simulink model "sgMdl_BMTS_SimpleVoltageControlWithBCE"  (R2024b)
settings: Solver=FixedStepAuto  StartTime=0.0  StopTime=inf  RelTol=1e-3  EnableMultiTasking=on
undefined symbols (not defined in the file): BCE12, BCE_Set_init, Device_01, sg_bce
libraries: slrealtimeethercatlib x99, simulink x13, slrealtimeutilitieslib x12, SignalEditorBlockLib x1
Description:
  | BMTS - Simple Voltage Control with BCE
settings Model: ModifiedByFormat=Speedgoat  SimulationMode=external  ExtModeTrigDuration=100000  Creator=Speedgoat  LastModifiedBy=Speedgoat
settings SolverCC: ConcurrentTasks=on  AlgebraicLoopSolver=TrustRegion  PositivePriorityOrder=on  InsertRTBMode=Never (minimum delay)
settings DataIOCC: SaveFormat=Array  SaveState=on  SignalLoggingName=logsOut
settings OptimizationCC: BlockReduction=off  BooleanDataType=off  OptimizeBlockIOStorage=off  BufferReuse=off  ReuseModelBlockBuffer=off  GlobalBufferReuse=off  ExpressionFolding=off  LocalBlockOutputs=off  InitFltsAndDblsToZero=on  OptimizeDataStoreBuffers=off  BusAssignmentInplaceUpdate=off
settings DebuggingCC: SaveWithParameterizedLinksMsg=none  MergeDetectMultiDrivingBlocksExec=none  CheckExecutionContextPreStartOutputMsg=on  SignalResolutionControl=TryResolveAllWithWarning  TasksWithSamePriorityMsg=none  UnconnectedInputMsg=warning  UnconnectedOutputMsg=warning  UnconnectedLineMsg=warning  SFUnexpectedBacktrackingDiag=warning  SFNoUnconditionalDefaultTransitionDiag=warning  SFExecutionAtInitializationDiag=none  ArithmeticOperatorsInVariantConditions=warning
settings HardwareCC: ProdBitPerLong=64  ProdLongLongMode=on  ProdHWDeviceType=Intel->x86-64 (Linux 64)
settings ModelReferenceCC: EnableRefExpFcnMdlSchedulingChecks=on  PropagateSignalLabelsOutOfModel=off
settings SFSimCC: SimUseLocalCustomCode=off  SimTargetLang=C++
settings RTWCC: Description=Speedgoat Real-Time Target Machine  SystemTargetFile=speedgoat.tlc  TemplateMakefile=slrealtime_default_tmf  RTWUseLocalCustomCode=off  Toolchain=Simulink Real-Time Toolchain  BuildConfiguration=Faster Runs  TargetLang=C++  GPUComputeCapability=3.5  DLArmComputeVersion=19.05
settings CodeAppCC: StateflowObjectComments=on
settings SimulinkRealTimeTargetCC: SubcomponentCodeInterfacePackaging=Reusable function  InstructionSetFMA=off  LogToMDFFile=off  SLRTFileLogMaxRuns=10
settings ConfigComp: CovMetricSettings=dw  CovSaveCumulativeToWorkspaceVar=on  CovSaveSingleToWorkspaceVar=on  CovExternalEMLEnable=off  CovSFcnEnable=off  CovBoundaryAbsTol=1.0e-5

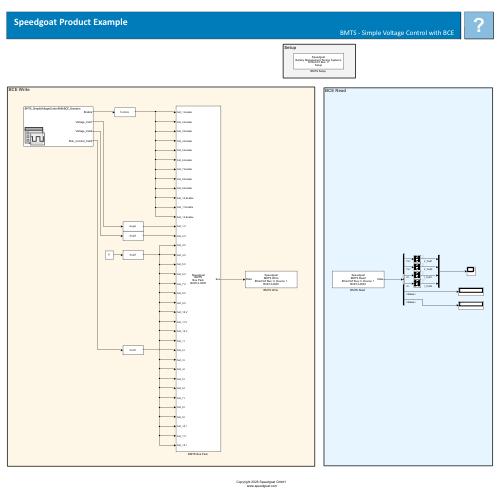
[thumbnail: Simulink's stored preview of the top-level diagram]
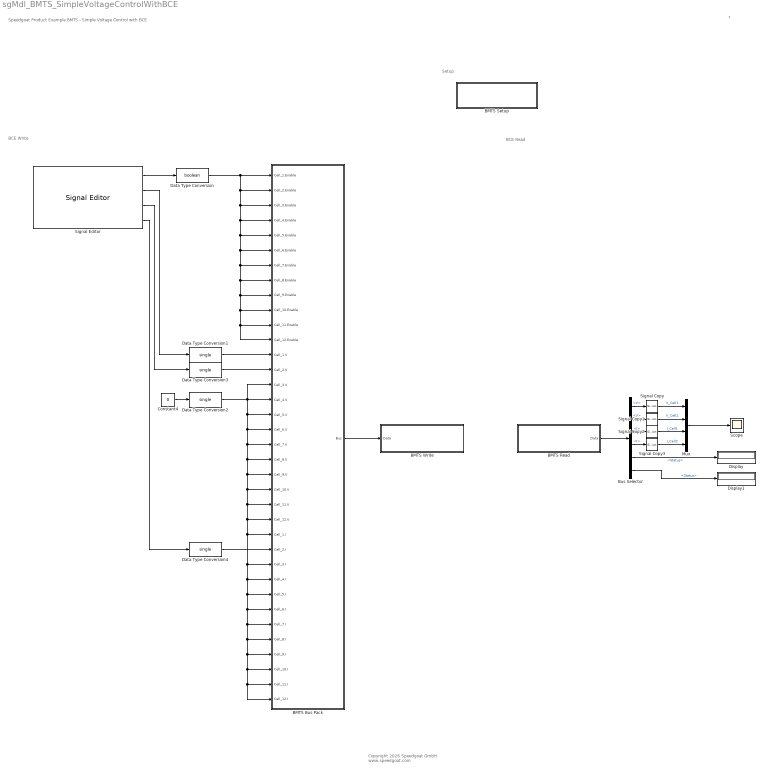
== system sgMdl_BMTS_SimpleVoltageControlWithBCE ==
  note: Setup
  note: BCE Write
  note: BCE Read
  note: Speedgoat Product Example
      | BMTS - Simple Voltage Control with BCE
  note: ?
  note: Copyright 2026 Speedgoat GmbH
      |  www.speedgoat.com
  "BMTS Bus Pack " : Subsystem  mask(bmts_bus_pack){}
      settings: OpenFcn=sg_bce.openFcnBuspack;
      mask Help: eval('sg.utils.help.show(''io_main/refentry_bmts_buspack'');')
      mask Display: disp('Speedgoat\nBMTS\nBus Pack\nBCE12-0605');
  "BMTS Read " : Subsystem  InitFcn=sg_bce.checkNumberOfBlocksGlobal(bdroot);  mask(bce_read){}
      settings: OpenFcn=sg_bce.openFcnRead;
      mask Help: eval('sg.utils.help.show(''io_main/refentry_bce_read'');')
      mask Display: disp('Speedgoat\nBMTS Read\nEtherCAT Bus: 0, Device: 1\nBCE12-0605');port_label('output',1,'Data');
  "BMTS Setup " : Subsystem  LoadFcn=|  InitFcn=|  mask(bce_setup){}
      LoadFcn=|
      | sg_bce.createBusSignals;
      | sg_bce.setupEniCallback(gcb, bdroot);
      InitFcn=|
      | sg_bce.createBusSignals;
      | sg_bce.checkNumberOfBlocksGlobal(bdroot);
      | sg_bce.setupEniCallback(gcb, bdroot);
      settings: OpenFcn=sg_bce.openFcnSetup;
      mask Help: eval('sg.utils.help.show(''io_main/refentry_bce_setup'');')
      mask Display: disp('Speedgoat\nBattery Management Testing Systems\nEtherCAT Bus: 0\nSetup');
  "BMTS Write " : Subsystem  InitFcn=sg_bce.checkNumberOfBlocksGlobal(bdroot);  mask(bce_write){}
      settings: OpenFcn=sg_bce.openFcnWrite;
      mask Help: eval('sg.utils.help.show(''io_main/refentry_bce_write'');')
      mask Display: disp('Speedgoat\nBMTS Write\nEtherCAT Bus: 0, Device: 1\nBCE12-0605');port_label('input',1,'Data');
  Bus Selector : BusSelector  OutputSignals=Cell_1.V,Cell_2.V,Cell_1.I,Cell_2.I,Cell_1.Status,Cell_2.Status
  Constant4 : Constant  Value=0
  Data Type Conversion : DataTypeConversion  OutDataTypeStr=boolean  SaturateOnIntegerOverflow=off  RndMeth=Floor
  Data Type Conversion{1..4} (4 alike) : DataTypeConversion  OutDataTypeStr=single  SaturateOnIntegerOverflow=off  RndMeth=Floor
  Display : Display
  Display1 : Display
  Mux : Mux
  Scope : Scope
  Signal Copy{,1..3} (4 alike) : SignalConversion  OverrideOpt=off
  Signal Editor : SignalEditorBlockLib/Signal Editor  FileName=BMTS_SimpleVoltageControlWithBCE_Scenario.mat  ActiveScenario=BMTS_SimpleVoltageControlWithBCE_Scenario  ActiveSignal=Voltage_Cell2  IsBus=off  OutputBusObjectStr=Bus: BusObject  SampleTime=0  ZeroCross=off  OutputAfterFinalValue=Setting to zero  Unit=inherit  PreserveSignalName=on  ApplySigPropsToAllScenarios=on  ApplySigPropsToAllSignals=off
  wires:
  Signal Editor/2 -> Data Type Conversion1/1
  "BMTS Bus Pack "/1(Bus) -> "BMTS Write "/1(Data)
  Signal Editor/1 -> Data Type Conversion/1
  "BMTS Read "/1(Data) -> Bus Selector/1
  Data Type Conversion/1 -> "BMTS Bus Pack "/11(Cell_11.Enable), "BMTS Bus Pack "/12(Cell_12.Enable), "BMTS Bus Pack "/10(Cell_10.Enable), "BMTS Bus Pack "/9(Cell_9.Enable), "BMTS Bus Pack "/8(Cell_8.Enable), "BMTS Bus Pack "/7(Cell_7.Enable), "BMTS Bus Pack "/6(Cell_6.Enable), "BMTS Bus Pack "/5(Cell_5.Enable), "BMTS Bus Pack "/4(Cell_4.Enable), "BMTS Bus Pack "/3(Cell_3.Enable), "BMTS Bus Pack "/2(Cell_2.Enable), "BMTS Bus Pack "/1(Cell_1.Enable)
  Constant4/1 -> Data Type Conversion2/1
  Data Type Conversion1/1 -> "BMTS Bus Pack "/13(Cell_1.V)
  Data Type Conversion2/1 -> "BMTS Bus Pack "/35(Cell_11.I), "BMTS Bus Pack "/36(Cell_12.I), "BMTS Bus Pack "/34(Cell_10.I), "BMTS Bus Pack "/33(Cell_9.I), "BMTS Bus Pack "/32(Cell_8.I), "BMTS Bus Pack "/31(Cell_7.I), "BMTS Bus Pack "/30(Cell_6.I), "BMTS Bus Pack "/29(Cell_5.I), "BMTS Bus Pack "/28(Cell_4.I), "BMTS Bus Pack "/27(Cell_3.I), "BMTS Bus Pack "/25(Cell_1.I), "BMTS Bus Pack "/24(Cell_12.V), "BMTS Bus Pack "/23(Cell_11.V), "BMTS Bus Pack "/22(Cell_10.V), "BMTS Bus Pack "/21(Cell_9.V), "BMTS Bus Pack "/20(Cell_8.V), "BMTS Bus Pack "/19(Cell_7.V), "BMTS Bus Pack "/18(Cell_6.V), "BMTS Bus Pack "/17(Cell_5.V), "BMTS Bus Pack "/16(Cell_4.V), "BMTS Bus Pack "/15(Cell_3.V)
  Bus Selector/1 -> Signal Copy/1  "<V>"
  Bus Selector/2 -> Signal Copy1/1  "<V>"
  Bus Selector/3 -> Signal Copy2/1  "<I>"
  Bus Selector/4 -> Signal Copy3/1  "<I>"
  Bus Selector/5 -> Display/1  "<Status>"
  Bus Selector/6 -> Display1/1  "<Status>"
  Signal Copy/1 -> Mux/1  "V_Cell1"
  Signal Copy1/1 -> Mux/2  "V_Cell2"
  Signal Copy2/1 -> Mux/3  "I_Cell1"
  Signal Copy3/1 -> Mux/4  "I_Cell2"
  Data Type Conversion3/1 -> "BMTS Bus Pack "/14(Cell_2.V)
  Signal Editor/3 -> Data Type Conversion3/1
  Signal Editor/4 -> Data Type Conversion4/1
  Data Type Conversion4/1 -> "BMTS Bus Pack "/26(Cell_2.I)
  Mux/1 -> Scope/1

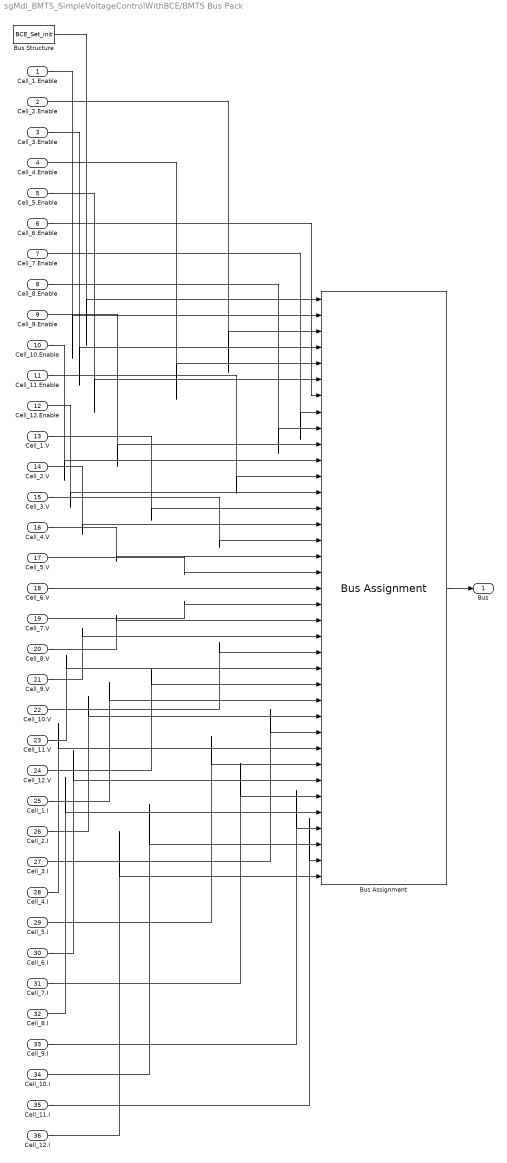
== system sgMdl_BMTS_SimpleVoltageControlWithBCE/BMTS Bus Pack  ==
  Cell_1.Enable : Inport
  Cell_2.Enable : Inport  Port=2
  Cell_3.Enable : Inport  Port=3
  Cell_4.Enable : Inport  Port=4
  Cell_5.Enable : Inport  Port=5
  Cell_6.Enable : Inport  Port=6
  Cell_7.Enable : Inport  Port=7
  Cell_8.Enable : Inport  Port=8
  Cell_9.Enable : Inport  Port=9
  Cell_10.Enable : Inport  Port=10
  Cell_11.Enable : Inport  Port=11
  Cell_12.Enable : Inport  Port=12
  Cell_1.V : Inport  Port=13
  Cell_2.V : Inport  Port=14
  Cell_3.V : Inport  Port=15
  Cell_4.V : Inport  Port=16
  Cell_5.V : Inport  Port=17
  Cell_6.V : Inport  Port=18
  Cell_7.V : Inport  Port=19
  Cell_8.V : Inport  Port=20
  Cell_9.V : Inport  Port=21
  Cell_10.V : Inport  Port=22
  Cell_11.V : Inport  Port=23
  Cell_12.V : Inport  Port=24
  Cell_1.I : Inport  Port=25
  Cell_2.I : Inport  Port=26
  Cell_3.I : Inport  Port=27
  Cell_4.I : Inport  Port=28
  Cell_5.I : Inport  Port=29
  Cell_6.I : Inport  Port=30
  Cell_7.I : Inport  Port=31
  Cell_8.I : Inport  Port=32
  Cell_9.I : Inport  Port=33
  Cell_10.I : Inport  Port=34
  Cell_11.I : Inport  Port=35
  Cell_12.I : Inport  Port=36
  Bus Assignment : BusAssignment  AssignedSignals=Cell_1.Enable,Cell_2.Enable,Cell_3.Enable,Cell_4.Enable,Cell_5.Enable,Cell_6.Enable,Cell_7.Enable,Cell_8.Enable,Cell_9.Enable,Cell_10.Enable,Cell_11.Enable,Cell_12.Enable,Cell_1.V,Cell_2.V,Cell_3.V,Cell_4.V,Cell_5.V,Cell_6.V,Cell_7.V,Cell_8.V,Cell_9.V,Cell_10.V,Cell_11.V,Cell_12.V,Cell_1.I,Cell_2.I,Cell_3.I,Cell_4.I,Cell_5.I,Cell_6.I,Cell_7.I,Cell_8.I,Cell_9.I,Cell_10.I,Cell_11.I,Cell_12.I
  Bus Structure : Constant  Value=BCE_Set_init  OutDataTypeStr=Bus: BCE_Set
  Bus : Outport
  wires:
  Cell_3.Enable/1 -> Bus Assignment/4
  Cell_5.Enable/1 -> Bus Assignment/6
  Cell_1.I/1 -> Bus Assignment/26
  Bus Structure/1 -> Bus Assignment/1
  Cell_1.Enable/1 -> Bus Assignment/2
  Cell_8.I/1 -> Bus Assignment/33
  Cell_7.Enable/1 -> Bus Assignment/8
  Cell_9.I/1 -> Bus Assignment/34
  Cell_2.Enable/1 -> Bus Assignment/3
  Cell_5.V/1 -> Bus Assignment/18
  Cell_4.Enable/1 -> Bus Assignment/5
  Cell_3.V/1 -> Bus Assignment/16
  Cell_8.Enable/1 -> Bus Assignment/9
  Cell_6.Enable/1 -> Bus Assignment/7
  Cell_6.I/1 -> Bus Assignment/31
  Cell_9.Enable/1 -> Bus Assignment/10
  Cell_10.Enable/1 -> Bus Assignment/11
  Cell_11.Enable/1 -> Bus Assignment/12
  Cell_11.I/1 -> Bus Assignment/36
  Cell_12.Enable/1 -> Bus Assignment/13
  Cell_1.V/1 -> Bus Assignment/14
  Cell_2.V/1 -> Bus Assignment/15
  Cell_12.V/1 -> Bus Assignment/25
  Cell_4.V/1 -> Bus Assignment/17
  Cell_6.V/1 -> Bus Assignment/19
  Cell_7.V/1 -> Bus Assignment/20
  Cell_3.I/1 -> Bus Assignment/28
  Cell_8.V/1 -> Bus Assignment/21
  Cell_9.V/1 -> Bus Assignment/22
  Cell_10.V/1 -> Bus Assignment/23
  Cell_11.V/1 -> Bus Assignment/24
  Cell_2.I/1 -> Bus Assignment/27
  Cell_4.I/1 -> Bus Assignment/29
  Cell_5.I/1 -> Bus Assignment/30
  Cell_7.I/1 -> Bus Assignment/32
  Cell_10.I/1 -> Bus Assignment/35
  Cell_12.I/1 -> Bus Assignment/37
  Bus Assignment/1 -> Bus/1

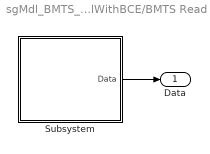
== system sgMdl_BMTS_SimpleVoltageControlWithBCE/BMTS Read  ==
  Subsystem : Subsystem
  Data : Outport  OutDataTypeStr=Bus: BCE_Get
  wires:
  Subsystem/1(Data) -> Data/1

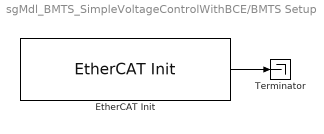
== system sgMdl_BMTS_SimpleVoltageControlWithBCE/BMTS Setup  ==
  EtherCAT Init : slrealtimeethercatlib/EtherCAT Init  Priority=0  config_file=C:\Users\timo.straessle\AppData\Local\Temp\sg_bmts\sgMdl_BMTS_SimpleVoltageControlWithBCE\sg_bmts_ENI_bus0.xml  device_id=0  portnum=1  initstate=2  dctuning=0  enaDebug=0  logFile='c:\dbglog.txt'  sample_time=0.001000  DCMode=0
  Terminator : Terminator
  wires:
  EtherCAT Init/1 -> Terminator/1

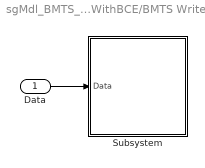
== system sgMdl_BMTS_SimpleVoltageControlWithBCE/BMTS Write  ==
  Data : Inport  OutDataTypeStr=Bus: BCE_Set
  Subsystem : Subsystem
  wires:
  Data/1 -> Subsystem/1(Data)

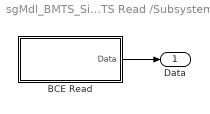
== system sgMdl_BMTS_SimpleVoltageControlWithBCE/BMTS Read /Subsystem ==
  "BCE Read " : Subsystem
  Data : Outport  OutDataTypeStr=Bus: BCE_Get
  wires:
  "BCE Read "/1(Data) -> Data/1

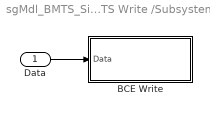
== system sgMdl_BMTS_SimpleVoltageControlWithBCE/BMTS Write /Subsystem ==
  Data : Inport  OutDataTypeStr=Bus: BCE_Set
  "BCE Write " : Subsystem
  wires:
  Data/1 -> "BCE Write "/1(Data)

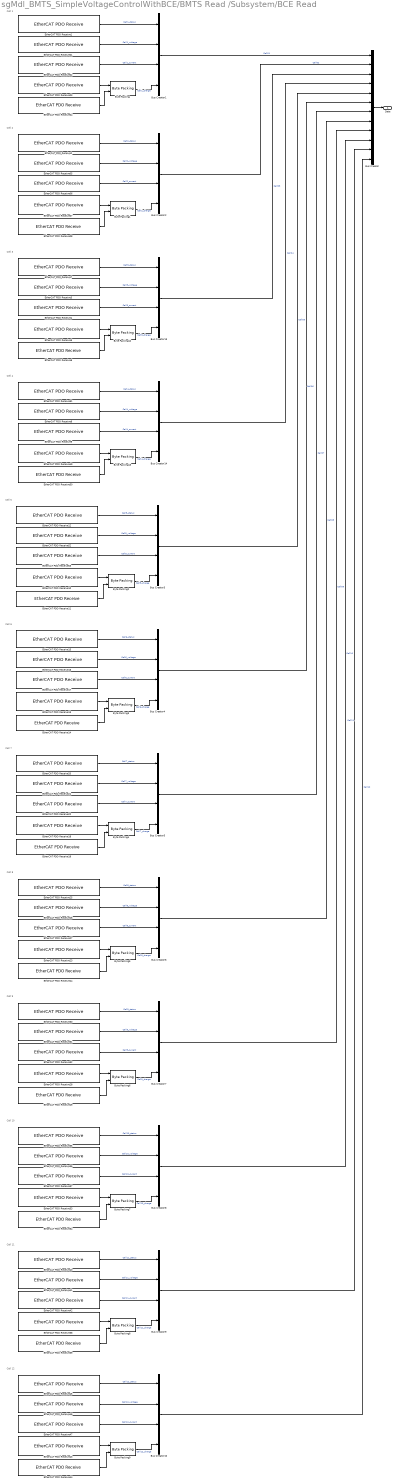
== system sgMdl_BMTS_SimpleVoltageControlWithBCE/BMTS Read /Subsystem/BCE Read  ==
  note: Cell 7
  note: Cell 2
  note: Cell 6
  note: Cell 8
  note: Cell 12
  note: Cell 11
  note: Cell 3
  note: Cell 5
  note: Cell 4
  note: Cell 10
  note: Cell 9
  note: Cell 1
  Bus Creator : BusCreator  Inputs=12  OutDataTypeStr=Bus: BCE_Get
      settings: InheritFromInputs=off
  Bus Creator{1..10,13..14} (12 alike) : BusCreator  Inputs=4  OutDataTypeStr=Bus: Cell_Get
      settings: InheritFromInputs=off
  Byte Packing{,1..9,12..13} (12 alike) : slrealtimeutilitieslib/Byte Packing  MaskPackedDataType=uint64  MaskUnpackedDataTypes={'uint32','uint32'}  MaskAlignment=1
  EtherCAT PDO Receive01 : slrealtimeethercatlib/EtherCAT PDO Receive  Priority=2  sig_name=Device_01 (BCE12-0605).Tx_Cell_01.voltage  sig_offset=16  sig_type=single  type_size=32  sig_dim=1  device_id=0  sample_time=0.001000
  EtherCAT PDO Receive02 : slrealtimeethercatlib/EtherCAT PDO Receive  Priority=2  sig_name=Device_01 (BCE12-0605).Tx_Cell_01.current  sig_offset=48  sig_type=single  type_size=32  sig_dim=1  device_id=0  sample_time=0.001000
  EtherCAT PDO Receive03 : slrealtimeethercatlib/EtherCAT PDO Receive  Priority=2  sig_name=Device_01 (BCE12-0605).Tx_Cell_01.chargeMSB  sig_offset=80  sig_type=uint32  type_size=32  sig_dim=1  device_id=0  sample_time=0.001000
  EtherCAT PDO Receive04 : slrealtimeethercatlib/EtherCAT PDO Receive  Priority=2  sig_name=Device_01 (BCE12-0605).Tx_Cell_01.chargeLSB  sig_offset=112  sig_type=uint32  type_size=32  sig_dim=1  device_id=0  sample_time=0.001000
  EtherCAT PDO Receive05 : slrealtimeethercatlib/EtherCAT PDO Receive  Priority=2  sig_name=Device_01 (BCE12-0605).Tx_Cell_02.voltage  sig_offset=160  sig_type=single  type_size=32  sig_dim=1  device_id=0  sample_time=0.001000
  EtherCAT PDO Receive06 : slrealtimeethercatlib/EtherCAT PDO Receive  Priority=2  sig_name=Device_01 (BCE12-0605).Tx_Cell_02.current  sig_offset=192  sig_type=single  type_size=32  sig_dim=1  device_id=0  sample_time=0.001000
  EtherCAT PDO Receive07 : slrealtimeethercatlib/EtherCAT PDO Receive  Priority=2  sig_name=Device_01 (BCE12-0605).Tx_Cell_02.chargeMSB  sig_offset=224  sig_type=uint32  type_size=32  sig_dim=1  device_id=0  sample_time=0.001000
  EtherCAT PDO Receive08 : slrealtimeethercatlib/EtherCAT PDO Receive  Priority=2  sig_name=Device_01 (BCE12-0605).Tx_Cell_02.chargeLSB  sig_offset=256  sig_type=uint32  type_size=32  sig_dim=1  device_id=0  sample_time=0.001000
  EtherCAT PDO Receive1 : slrealtimeethercatlib/EtherCAT PDO Receive  Priority=2  sig_name=Device_01 (BCE12-0605).Tx_Cell_01.status  sig_offset=0  sig_type=uint16  type_size=16  sig_dim=1  device_id=0  sample_time=0.001000
  EtherCAT PDO Receive10 : slrealtimeethercatlib/EtherCAT PDO Receive  Priority=2  sig_name=Device_01 (BCE12-0605).Tx_Cell_05.chargeMSB  sig_offset=656  sig_type=uint32  type_size=32  sig_dim=1  device_id=0  sample_time=0.001000
  EtherCAT PDO Receive11 : slrealtimeethercatlib/EtherCAT PDO Receive  Priority=2  sig_name=Device_01 (BCE12-0605).Tx_Cell_05.chargeLSB  sig_offset=688  sig_type=uint32  type_size=32  sig_dim=1  device_id=0  sample_time=0.001000
  EtherCAT PDO Receive12 : slrealtimeethercatlib/EtherCAT PDO Receive  Priority=2  sig_name=Device_01 (BCE12-0605).Tx_Cell_05.status  sig_offset=576  sig_type=uint16  type_size=16  sig_dim=1  device_id=0  sample_time=0.001000
  EtherCAT PDO Receive13 : slrealtimeethercatlib/EtherCAT PDO Receive  Priority=2  sig_name=Device_01 (BCE12-0605).Tx_Cell_06.chargeMSB  sig_offset=800  sig_type=uint32  type_size=32  sig_dim=1  device_id=0  sample_time=0.001000
  EtherCAT PDO Receive14 : slrealtimeethercatlib/EtherCAT PDO Receive  Priority=2  sig_name=Device_01 (BCE12-0605).Tx_Cell_06.chargeLSB  sig_offset=832  sig_type=uint32  type_size=32  sig_dim=1  device_id=0  sample_time=0.001000
  EtherCAT PDO Receive15 : slrealtimeethercatlib/EtherCAT PDO Receive  Priority=2  sig_name=Device_01 (BCE12-0605).Tx_Cell_06.status  sig_offset=720  sig_type=uint16  type_size=16  sig_dim=1  device_id=0  sample_time=0.001000
  EtherCAT PDO Receive16 : slrealtimeethercatlib/EtherCAT PDO Receive  Priority=2  sig_name=Device_01 (BCE12-0605).Tx_Cell_06.voltage  sig_offset=736  sig_type=single  type_size=32  sig_dim=1  device_id=0  sample_time=0.001000
  EtherCAT PDO Receive17 : slrealtimeethercatlib/EtherCAT PDO Receive  Priority=2  sig_name=Device_01 (BCE12-0605).Tx_Cell_06.current  sig_offset=768  sig_type=single  type_size=32  sig_dim=1  device_id=0  sample_time=0.001000
  EtherCAT PDO Receive18 : slrealtimeethercatlib/EtherCAT PDO Receive  Priority=2  sig_name=Device_01 (BCE12-0605).Tx_Cell_07.chargeMSB  sig_offset=944  sig_type=uint32  type_size=32  sig_dim=1  device_id=0  sample_time=0.001000
  EtherCAT PDO Receive19 : slrealtimeethercatlib/EtherCAT PDO Receive  Priority=2  sig_name=Device_01 (BCE12-0605).Tx_Cell_07.chargeLSB  sig_offset=976  sig_type=uint32  type_size=32  sig_dim=1  device_id=0  sample_time=0.001000
  EtherCAT PDO Receive2 : slrealtimeethercatlib/EtherCAT PDO Receive  Priority=2  sig_name=Device_01 (BCE12-0605).Tx_Cell_02.status  sig_offset=144  sig_type=uint16  type_size=16  sig_dim=1  device_id=0  sample_time=0.001000
  EtherCAT PDO Receive20 : slrealtimeethercatlib/EtherCAT PDO Receive  Priority=2  sig_name=Device_01 (BCE12-0605).Tx_Cell_07.status  sig_offset=864  sig_type=uint16  type_size=16  sig_dim=1  device_id=0  sample_time=0.001000
  EtherCAT PDO Receive21 : slrealtimeethercatlib/EtherCAT PDO Receive  Priority=2  sig_name=Device_01 (BCE12-0605).Tx_Cell_07.voltage  sig_offset=880  sig_type=single  type_size=32  sig_dim=1  device_id=0  sample_time=0.001000
  EtherCAT PDO Receive22 : slrealtimeethercatlib/EtherCAT PDO Receive  Priority=2  sig_name=Device_01 (BCE12-0605).Tx_Cell_07.current  sig_offset=912  sig_type=single  type_size=32  sig_dim=1  device_id=0  sample_time=0.001000
  EtherCAT PDO Receive23 : slrealtimeethercatlib/EtherCAT PDO Receive  Priority=2  sig_name=Device_01 (BCE12-0605).Tx_Cell_08.chargeMSB  sig_offset=1088  sig_type=uint32  type_size=32  sig_dim=1  device_id=0  sample_time=0.001000
  EtherCAT PDO Receive24 : slrealtimeethercatlib/EtherCAT PDO Receive  Priority=2  sig_name=Device_01 (BCE12-0605).Tx_Cell_08.chargeLSB  sig_offset=1120  sig_type=uint32  type_size=32  sig_dim=1  device_id=0  sample_time=0.001000
  EtherCAT PDO Receive25 : slrealtimeethercatlib/EtherCAT PDO Receive  Priority=2  sig_name=Device_01 (BCE12-0605).Tx_Cell_08.status  sig_offset=1008  sig_type=uint16  type_size=16  sig_dim=1  device_id=0  sample_time=0.001000
  EtherCAT PDO Receive26 : slrealtimeethercatlib/EtherCAT PDO Receive  Priority=2  sig_name=Device_01 (BCE12-0605).Tx_Cell_08.voltage  sig_offset=1024  sig_type=single  type_size=32  sig_dim=1  device_id=0  sample_time=0.001000
  EtherCAT PDO Receive27 : slrealtimeethercatlib/EtherCAT PDO Receive  Priority=2  sig_name=Device_01 (BCE12-0605).Tx_Cell_08.current  sig_offset=1056  sig_type=single  type_size=32  sig_dim=1  device_id=0  sample_time=0.001000
  EtherCAT PDO Receive28 : slrealtimeethercatlib/EtherCAT PDO Receive  Priority=2  sig_name=Device_01 (BCE12-0605).Tx_Cell_09.chargeMSB  sig_offset=1232  sig_type=uint32  type_size=32  sig_dim=1  device_id=0  sample_time=0.001000
  EtherCAT PDO Receive29 : slrealtimeethercatlib/EtherCAT PDO Receive  Priority=2  sig_name=Device_01 (BCE12-0605).Tx_Cell_09.chargeLSB  sig_offset=1264  sig_type=uint32  type_size=32  sig_dim=1  device_id=0  sample_time=0.001000
  EtherCAT PDO Receive3 : slrealtimeethercatlib/EtherCAT PDO Receive  Priority=2  sig_name=Device_01 (BCE12-0605).Tx_Cell_03.voltage  sig_offset=304  sig_type=single  type_size=32  sig_dim=1  device_id=0  sample_time=0.001000
  EtherCAT PDO Receive30 : slrealtimeethercatlib/EtherCAT PDO Receive  Priority=2  sig_name=Device_01 (BCE12-0605).Tx_Cell_09.status  sig_offset=1152  sig_type=uint16  type_size=16  sig_dim=1  device_id=0  sample_time=0.001000
  EtherCAT PDO Receive31 : slrealtimeethercatlib/EtherCAT PDO Receive  Priority=2  sig_name=Device_01 (BCE12-0605).Tx_Cell_09.voltage  sig_offset=1168  sig_type=single  type_size=32  sig_dim=1  device_id=0  sample_time=0.001000
  EtherCAT PDO Receive32 : slrealtimeethercatlib/EtherCAT PDO Receive  Priority=2  sig_name=Device_01 (BCE12-0605).Tx_Cell_09.current  sig_offset=1200  sig_type=single  type_size=32  sig_dim=1  device_id=0  sample_time=0.001000
  EtherCAT PDO Receive33 : slrealtimeethercatlib/EtherCAT PDO Receive  Priority=2  sig_name=Device_01 (BCE12-0605).Tx_Cell_10.chargeMSB  sig_offset=1376  sig_type=uint32  type_size=32  sig_dim=1  device_id=0  sample_time=0.001000
  EtherCAT PDO Receive34 : slrealtimeethercatlib/EtherCAT PDO Receive  Priority=2  sig_name=Device_01 (BCE12-0605).Tx_Cell_10.chargeLSB  sig_offset=1408  sig_type=uint32  type_size=32  sig_dim=1  device_id=0  sample_time=0.001000
  EtherCAT PDO Receive35 : slrealtimeethercatlib/EtherCAT PDO Receive  Priority=2  sig_name=Device_01 (BCE12-0605).Tx_Cell_10.status  sig_offset=1296  sig_type=uint16  type_size=16  sig_dim=1  device_id=0  sample_time=0.001000
  EtherCAT PDO Receive36 : slrealtimeethercatlib/EtherCAT PDO Receive  Priority=2  sig_name=Device_01 (BCE12-0605).Tx_Cell_10.voltage  sig_offset=1312  sig_type=single  type_size=32  sig_dim=1  device_id=0  sample_time=0.001000
  EtherCAT PDO Receive37 : slrealtimeethercatlib/EtherCAT PDO Receive  Priority=2  sig_name=Device_01 (BCE12-0605).Tx_Cell_10.current  sig_offset=1344  sig_type=single  type_size=32  sig_dim=1  device_id=0  sample_time=0.001000
  EtherCAT PDO Receive38 : slrealtimeethercatlib/EtherCAT PDO Receive  Priority=2  sig_name=Device_01 (BCE12-0605).Tx_Cell_11.chargeMSB  sig_offset=1520  sig_type=uint32  type_size=32  sig_dim=1  device_id=0  sample_time=0.001000
  EtherCAT PDO Receive39 : slrealtimeethercatlib/EtherCAT PDO Receive  Priority=2  sig_name=Device_01 (BCE12-0605).Tx_Cell_11.chargeLSB  sig_offset=1552  sig_type=uint32  type_size=32  sig_dim=1  device_id=0  sample_time=0.001000
  EtherCAT PDO Receive4 : slrealtimeethercatlib/EtherCAT PDO Receive  Priority=2  sig_name=Device_01 (BCE12-0605).Tx_Cell_03.current  sig_offset=336  sig_type=single  type_size=32  sig_dim=1  device_id=0  sample_time=0.001000
  EtherCAT PDO Receive40 : slrealtimeethercatlib/EtherCAT PDO Receive  Priority=2  sig_name=Device_01 (BCE12-0605).Tx_Cell_11.status  sig_offset=1440  sig_type=uint16  type_size=16  sig_dim=1  device_id=0  sample_time=0.001000
  EtherCAT PDO Receive41 : slrealtimeethercatlib/EtherCAT PDO Receive  Priority=2  sig_name=Device_01 (BCE12-0605).Tx_Cell_11.voltage  sig_offset=1456  sig_type=single  type_size=32  sig_dim=1  device_id=0  sample_time=0.001000
  EtherCAT PDO Receive42 : slrealtimeethercatlib/EtherCAT PDO Receive  Priority=2  sig_name=Device_01 (BCE12-0605).Tx_Cell_11.current  sig_offset=1488  sig_type=single  type_size=32  sig_dim=1  device_id=0  sample_time=0.001000
  EtherCAT PDO Receive43 : slrealtimeethercatlib/EtherCAT PDO Receive  Priority=2  sig_name=Device_01 (BCE12-0605).Tx_Cell_12.chargeMSB  sig_offset=1664  sig_type=uint32  type_size=32  sig_dim=1  device_id=0  sample_time=0.001000
  EtherCAT PDO Receive44 : slrealtimeethercatlib/EtherCAT PDO Receive  Priority=2  sig_name=Device_01 (BCE12-0605).Tx_Cell_12.chargeLSB  sig_offset=1696  sig_type=uint32  type_size=32  sig_dim=1  device_id=0  sample_time=0.001000
  EtherCAT PDO Receive45 : slrealtimeethercatlib/EtherCAT PDO Receive  Priority=2  sig_name=Device_01 (BCE12-0605).Tx_Cell_12.status  sig_offset=1584  sig_type=uint16  type_size=16  sig_dim=1  device_id=0  sample_time=0.001000
  EtherCAT PDO Receive46 : slrealtimeethercatlib/EtherCAT PDO Receive  Priority=2  sig_name=Device_01 (BCE12-0605).Tx_Cell_12.voltage  sig_offset=1600  sig_type=single  type_size=32  sig_dim=1  device_id=0  sample_time=0.001000
  EtherCAT PDO Receive47 : slrealtimeethercatlib/EtherCAT PDO Receive  Priority=2  sig_name=Device_01 (BCE12-0605).Tx_Cell_12.current  sig_offset=1632  sig_type=single  type_size=32  sig_dim=1  device_id=0  sample_time=0.001000
  EtherCAT PDO Receive49 : slrealtimeethercatlib/EtherCAT PDO Receive  Priority=2  sig_name=Device_01 (BCE12-0605).Tx_Cell_04.chargeMSB  sig_offset=512  sig_type=uint32  type_size=32  sig_dim=1  device_id=0  sample_time=0.001000
  EtherCAT PDO Receive5 : slrealtimeethercatlib/EtherCAT PDO Receive  Priority=2  sig_name=Device_01 (BCE12-0605).Tx_Cell_03.chargeMSB  sig_offset=368  sig_type=uint32  type_size=32  sig_dim=1  device_id=0  sample_time=0.001000
  EtherCAT PDO Receive50 : slrealtimeethercatlib/EtherCAT PDO Receive  Priority=2  sig_name=Device_01 (BCE12-0605).Tx_Cell_04.chargeLSB  sig_offset=544  sig_type=uint32  type_size=32  sig_dim=1  device_id=0  sample_time=0.001000
  EtherCAT PDO Receive51 : slrealtimeethercatlib/EtherCAT PDO Receive  Priority=2  sig_name=Device_01 (BCE12-0605).Tx_Cell_04.status  sig_offset=432  sig_type=uint16  type_size=16  sig_dim=1  device_id=0  sample_time=0.001000
  EtherCAT PDO Receive52 : slrealtimeethercatlib/EtherCAT PDO Receive  Priority=2  sig_name=Device_01 (BCE12-0605).Tx_Cell_05.voltage  sig_offset=592  sig_type=single  type_size=32  sig_dim=1  device_id=0  sample_time=0.001000
  EtherCAT PDO Receive53 : slrealtimeethercatlib/EtherCAT PDO Receive  Priority=2  sig_name=Device_01 (BCE12-0605).Tx_Cell_05.current  sig_offset=624  sig_type=single  type_size=32  sig_dim=1  device_id=0  sample_time=0.001000
  EtherCAT PDO Receive6 : slrealtimeethercatlib/EtherCAT PDO Receive  Priority=2  sig_name=Device_01 (BCE12-0605).Tx_Cell_03.chargeLSB  sig_offset=400  sig_type=uint32  type_size=32  sig_dim=1  device_id=0  sample_time=0.001000
  EtherCAT PDO Receive7 : slrealtimeethercatlib/EtherCAT PDO Receive  Priority=2  sig_name=Device_01 (BCE12-0605).Tx_Cell_03.status  sig_offset=288  sig_type=uint16  type_size=16  sig_dim=1  device_id=0  sample_time=0.001000
  EtherCAT PDO Receive8 : slrealtimeethercatlib/EtherCAT PDO Receive  Priority=2  sig_name=Device_01 (BCE12-0605).Tx_Cell_04.voltage  sig_offset=448  sig_type=single  type_size=32  sig_dim=1  device_id=0  sample_time=0.001000
  EtherCAT PDO Receive9 : slrealtimeethercatlib/EtherCAT PDO Receive  Priority=2  sig_name=Device_01 (BCE12-0605).Tx_Cell_04.current  sig_offset=480  sig_type=single  type_size=32  sig_dim=1  device_id=0  sample_time=0.001000
  Data : Outport  OutDataTypeStr=Bus: BCE_Get
  wires:
  EtherCAT PDO Receive04/1 -> Byte Packing/2
  EtherCAT PDO Receive53/1 -> Bus Creator3/3  "Cell5_current"
  Bus Creator7/1 -> Bus Creator/9  "Cell09"
  EtherCAT PDO Receive1/1 -> Bus Creator1/1  "Cell1_status"
  EtherCAT PDO Receive40/1 -> Bus Creator9/1  "Cell11_status"
  EtherCAT PDO Receive39/1 -> Byte Packing8/2
  EtherCAT PDO Receive18/1 -> Byte Packing4/1
  Byte Packing13/1 -> Bus Creator14/4  "Cell4_charge"
  Bus Creator14/1 -> Bus Creator/4  "Cell04"
  EtherCAT PDO Receive21/1 -> Bus Creator5/2  "Cell7_voltage"
  EtherCAT PDO Receive52/1 -> Bus Creator3/2  "Cell5_voltage"
  EtherCAT PDO Receive15/1 -> Bus Creator4/1  "Cell6_status"
  EtherCAT PDO Receive11/1 -> Byte Packing2/2
  EtherCAT PDO Receive26/1 -> Bus Creator6/2  "Cell8_voltage"
  EtherCAT PDO Receive33/1 -> Byte Packing7/1
  EtherCAT PDO Receive12/1 -> Bus Creator3/1  "Cell5_status"
  Byte Packing2/1 -> Bus Creator3/4  "Cell5_charge"
  Byte Packing4/1 -> Bus Creator5/4  "Cell7_charge"
  Byte Packing6/1 -> Bus Creator7/4  "Cell9_charge"
  EtherCAT PDO Receive7/1 -> Bus Creator13/1  "Cell3_status"
  Bus Creator4/1 -> Bus Creator/6  "Cell06"
  Bus Creator6/1 -> Bus Creator/8  "Cell08"
  EtherCAT PDO Receive30/1 -> Bus Creator7/1  "Cell9_status"
  EtherCAT PDO Receive4/1 -> Bus Creator13/3  "Cell3_current"
  Bus Creator13/1 -> Bus Creator/3  "Cell03"
  Byte Packing7/1 -> Bus Creator8/4  "Cell10_charge"
  EtherCAT PDO Receive01/1 -> Bus Creator1/2  "Cell1_voltage"
  EtherCAT PDO Receive35/1 -> Bus Creator8/1  "Cell10_status"
  EtherCAT PDO Receive29/1 -> Byte Packing6/2
  EtherCAT PDO Receive27/1 -> Bus Creator6/3  "Cell8_current"
  EtherCAT PDO Receive32/1 -> Bus Creator7/3  "Cell9_current"
  EtherCAT PDO Receive41/1 -> Bus Creator9/2  "Cell11_voltage"
  EtherCAT PDO Receive5/1 -> Byte Packing12/1
  EtherCAT PDO Receive3/1 -> Bus Creator13/2  "Cell3_voltage"
  EtherCAT PDO Receive46/1 -> Bus Creator10/2  "Cell12_voltage"
  EtherCAT PDO Receive6/1 -> Byte Packing12/2
  EtherCAT PDO Receive17/1 -> Bus Creator4/3  "Cell6_current"
  EtherCAT PDO Receive9/1 -> Bus Creator14/3  "Cell4_current"
  Bus Creator9/1 -> Bus Creator/11  "Cell11"
  EtherCAT PDO Receive43/1 -> Byte Packing9/1
  EtherCAT PDO Receive44/1 -> Byte Packing9/2
  EtherCAT PDO Receive45/1 -> Bus Creator10/1  "Cell12_status"
  EtherCAT PDO Receive23/1 -> Byte Packing5/1
  EtherCAT PDO Receive37/1 -> Bus Creator8/3  "Cell10_current"
  EtherCAT PDO Receive8/1 -> Bus Creator14/2  "Cell4_voltage"
  EtherCAT PDO Receive14/1 -> Byte Packing3/2
  EtherCAT PDO Receive49/1 -> Byte Packing13/1
  EtherCAT PDO Receive19/1 -> Byte Packing4/2
  EtherCAT PDO Receive24/1 -> Byte Packing5/2
  Bus Creator2/1 -> Bus Creator/2  "Cell02"
  Bus Creator5/1 -> Bus Creator/7  "Cell07"
  Byte Packing8/1 -> Bus Creator9/4  "Cell11_charge"
  Byte Packing1/1 -> Bus Creator2/4  "Cell2_charge"
  Bus Creator10/1 -> Bus Creator/12  "Cell12"
  Bus Creator8/1 -> Bus Creator/10  "Cell10"
  EtherCAT PDO Receive28/1 -> Byte Packing6/1
  Byte Packing3/1 -> Bus Creator4/4  "Cell6_charge"
  EtherCAT PDO Receive13/1 -> Byte Packing3/1
  EtherCAT PDO Receive16/1 -> Bus Creator4/2  "Cell6_voltage"
  EtherCAT PDO Receive51/1 -> Bus Creator14/1  "Cell4_status"
  EtherCAT PDO Receive05/1 -> Bus Creator2/2  "Cell2_voltage"
  EtherCAT PDO Receive06/1 -> Bus Creator2/3  "Cell2_current"
  EtherCAT PDO Receive25/1 -> Bus Creator6/1  "Cell8_status"
  EtherCAT PDO Receive31/1 -> Bus Creator7/2  "Cell9_voltage"
  Byte Packing12/1 -> Bus Creator13/4  "Cell3_charge"
  Byte Packing/1 -> Bus Creator1/4  "Cell1_charge"
  EtherCAT PDO Receive38/1 -> Byte Packing8/1
  EtherCAT PDO Receive50/1 -> Byte Packing13/2
  Bus Creator3/1 -> Bus Creator/5  "Cell05"
  EtherCAT PDO Receive22/1 -> Bus Creator5/3  "Cell7_current"
  Byte Packing9/1 -> Bus Creator10/4  "Cell12_charge"
  Byte Packing5/1 -> Bus Creator6/4  "Cell8_charge"
  Bus Creator1/1 -> Bus Creator/1  "Cell01"
  EtherCAT PDO Receive36/1 -> Bus Creator8/2  "Cell10_voltage"
  EtherCAT PDO Receive07/1 -> Byte Packing1/1
  EtherCAT PDO Receive47/1 -> Bus Creator10/3  "Cell12_current"
  EtherCAT PDO Receive10/1 -> Byte Packing2/1
  EtherCAT PDO Receive20/1 -> Bus Creator5/1  "Cell7_status"
  EtherCAT PDO Receive42/1 -> Bus Creator9/3  "Cell11_current"
  EtherCAT PDO Receive02/1 -> Bus Creator1/3  "Cell1_current"
  EtherCAT PDO Receive34/1 -> Byte Packing7/2
  EtherCAT PDO Receive2/1 -> Bus Creator2/1  "Cell2_status"
  Bus Creator/1 -> Data/1
  EtherCAT PDO Receive03/1 -> Byte Packing/1
  EtherCAT PDO Receive08/1 -> Byte Packing1/2

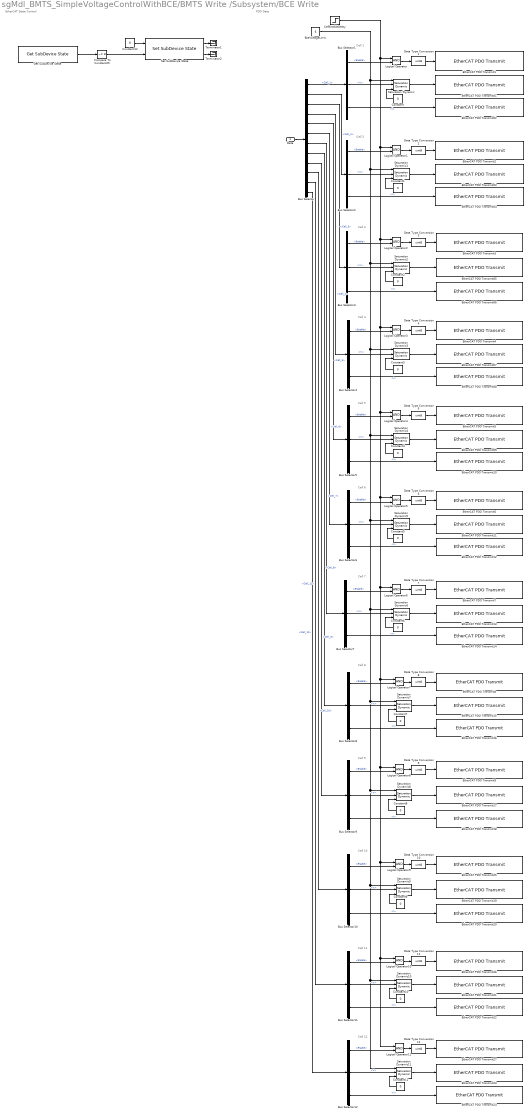
== system sgMdl_BMTS_SimpleVoltageControlWithBCE/BMTS Write /Subsystem/BCE Write  ==
  note: EtherCAT State Control
  note: Cell 4
  note: Cell 8
  note: Cell 9
  note: Cell 1
  note: Cell 7
  note: PDO Data
  note: Cell 5
  note: Cell 3
  note: Cell 10
  note: Cell 6
  note: Cell 11
  note: Cell 12
  note: Cell 2
  Data : Inport  OutDataTypeStr=Bus: BCE_Set
  BceVoltageLimit : Constant  Value=6  SampleTime=0.001
  Bus Selector : BusSelector  OutputSignals=Cell_1,Cell_2,Cell_3,Cell_4,Cell_5,Cell_6,Cell_7,Cell_8,Cell_9,Cell_10,Cell_11,Cell_12
  Bus Selector{1..12} (12 alike) : BusSelector  OutputSignals=Enable,V,I
  CellEnableDelay : Step  Time=2  SampleTime=0.001
  Compare To Constant25 : simulink/Logic and Bit Operations/Compare To Constant  relop=~=  const=8  OutDataTypeStr=boolean
  Constant{,1..11} (12 alike) : Constant  Value=0
  Constant12 : Constant  Value=8  OutDataTypeStr=int32
  Data Type Conversion{1..12} (12 alike) : DataTypeConversion  OutDataTypeStr=uint8  SaturateOnIntegerOverflow=off  RndMeth=Floor
  EtherCAT PDO Transmit01 : slrealtimeethercatlib/EtherCAT PDO Transmit  Priority=3  sig_name=Device_01 (BCE12-0605).Rx_Cell_01.setVoltage  sig_offset=8  sig_type=single  type_size=32  sig_dim=1  device_id=0  sample_time=0.001000
  EtherCAT PDO Transmit02 : slrealtimeethercatlib/EtherCAT PDO Transmit  Priority=3  sig_name=Device_01 (BCE12-0605).Rx_Cell_01.setCurrent  sig_offset=40  sig_type=single  type_size=32  sig_dim=1  device_id=0  sample_time=0.001000
  EtherCAT PDO Transmit03 : slrealtimeethercatlib/EtherCAT PDO Transmit  Priority=3  sig_name=Device_01 (BCE12-0605).Rx_Cell_02.setVoltage  sig_offset=80  sig_type=single  type_size=32  sig_dim=1  device_id=0  sample_time=0.001000
  EtherCAT PDO Transmit04 : slrealtimeethercatlib/EtherCAT PDO Transmit  Priority=3  sig_name=Device_01 (BCE12-0605).Rx_Cell_02.setCurrent  sig_offset=112  sig_type=single  type_size=32  sig_dim=1  device_id=0  sample_time=0.001000
  EtherCAT PDO Transmit05 : slrealtimeethercatlib/EtherCAT PDO Transmit  Priority=3  sig_name=Device_01 (BCE12-0605).Rx_Cell_03.setVoltage  sig_offset=152  sig_type=single  type_size=32  sig_dim=1  device_id=0  sample_time=0.001000
  EtherCAT PDO Transmit06 : slrealtimeethercatlib/EtherCAT PDO Transmit  Priority=3  sig_name=Device_01 (BCE12-0605).Rx_Cell_03.setCurrent  sig_offset=184  sig_type=single  type_size=32  sig_dim=1  device_id=0  sample_time=0.001000
  EtherCAT PDO Transmit07 : slrealtimeethercatlib/EtherCAT PDO Transmit  Priority=3  sig_name=Device_01 (BCE12-0605).Rx_Cell_04.setVoltage  sig_offset=224  sig_type=single  type_size=32  sig_dim=1  device_id=0  sample_time=0.001000
  EtherCAT PDO Transmit08 : slrealtimeethercatlib/EtherCAT PDO Transmit  Priority=3  sig_name=Device_01 (BCE12-0605).Rx_Cell_04.setCurrent  sig_offset=256  sig_type=single  type_size=32  sig_dim=1  device_id=0  sample_time=0.001000
  EtherCAT PDO Transmit09 : slrealtimeethercatlib/EtherCAT PDO Transmit  Priority=3  sig_name=Device_01 (BCE12-0605).Rx_Cell_05.setVoltage  sig_offset=296  sig_type=single  type_size=32  sig_dim=1  device_id=0  sample_time=0.001000
  EtherCAT PDO Transmit1 : slrealtimeethercatlib/EtherCAT PDO Transmit  Priority=3  sig_name=Device_01 (BCE12-0605).Rx_Cell_01.enableCell  sig_offset=0  sig_type=uint8  type_size=8  sig_dim=1  device_id=0  sample_time=0.001000
  EtherCAT PDO Transmit10 : slrealtimeethercatlib/EtherCAT PDO Transmit  Priority=3  sig_name=Device_01 (BCE12-0605).Rx_Cell_05.setCurrent  sig_offset=328  sig_type=single  type_size=32  sig_dim=1  device_id=0  sample_time=0.001000
  EtherCAT PDO Transmit11 : slrealtimeethercatlib/EtherCAT PDO Transmit  Priority=3  sig_name=Device_01 (BCE12-0605).Rx_Cell_06.setVoltage  sig_offset=368  sig_type=single  type_size=32  sig_dim=1  device_id=0  sample_time=0.001000
  EtherCAT PDO Transmit12 : slrealtimeethercatlib/EtherCAT PDO Transmit  Priority=3  sig_name=Device_01 (BCE12-0605).Rx_Cell_06.setCurrent  sig_offset=400  sig_type=single  type_size=32  sig_dim=1  device_id=0  sample_time=0.001000
  EtherCAT PDO Transmit13 : slrealtimeethercatlib/EtherCAT PDO Transmit  Priority=3  sig_name=Device_01 (BCE12-0605).Rx_Cell_07.setVoltage  sig_offset=440  sig_type=single  type_size=32  sig_dim=1  device_id=0  sample_time=0.001000
  EtherCAT PDO Transmit14 : slrealtimeethercatlib/EtherCAT PDO Transmit  Priority=3  sig_name=Device_01 (BCE12-0605).Rx_Cell_07.setCurrent  sig_offset=472  sig_type=single  type_size=32  sig_dim=1  device_id=0  sample_time=0.001000
  EtherCAT PDO Transmit15 : slrealtimeethercatlib/EtherCAT PDO Transmit  Priority=3  sig_name=Device_01 (BCE12-0605).Rx_Cell_08.setVoltage  sig_offset=512  sig_type=single  type_size=32  sig_dim=1  device_id=0  sample_time=0.001000
  EtherCAT PDO Transmit16 : slrealtimeethercatlib/EtherCAT PDO Transmit  Priority=3  sig_name=Device_01 (BCE12-0605).Rx_Cell_08.setCurrent  sig_offset=544  sig_type=single  type_size=32  sig_dim=1  device_id=0  sample_time=0.001000
  EtherCAT PDO Transmit17 : slrealtimeethercatlib/EtherCAT PDO Transmit  Priority=3  sig_name=Device_01 (BCE12-0605).Rx_Cell_09.setVoltage  sig_offset=584  sig_type=single  type_size=32  sig_dim=1  device_id=0  sample_time=0.001000
  EtherCAT PDO Transmit18 : slrealtimeethercatlib/EtherCAT PDO Transmit  Priority=3  sig_name=Device_01 (BCE12-0605).Rx_Cell_09.setCurrent  sig_offset=616  sig_type=single  type_size=32  sig_dim=1  device_id=0  sample_time=0.001000
  EtherCAT PDO Transmit19 : slrealtimeethercatlib/EtherCAT PDO Transmit  Priority=3  sig_name=Device_01 (BCE12-0605).Rx_Cell_10.setVoltage  sig_offset=656  sig_type=single  type_size=32  sig_dim=1  device_id=0  sample_time=0.001000
  EtherCAT PDO Transmit2 : slrealtimeethercatlib/EtherCAT PDO Transmit  Priority=3  sig_name=Device_01 (BCE12-0605).Rx_Cell_02.enableCell  sig_offset=72  sig_type=uint8  type_size=8  sig_dim=1  device_id=0  sample_time=0.001000
  EtherCAT PDO Transmit20 : slrealtimeethercatlib/EtherCAT PDO Transmit  Priority=3  sig_name=Device_01 (BCE12-0605).Rx_Cell_10.setCurrent  sig_offset=688  sig_type=single  type_size=32  sig_dim=1  device_id=0  sample_time=0.001000
  EtherCAT PDO Transmit21 : slrealtimeethercatlib/EtherCAT PDO Transmit  Priority=3  sig_name=Device_01 (BCE12-0605).Rx_Cell_11.setVoltage  sig_offset=728  sig_type=single  type_size=32  sig_dim=1  device_id=0  sample_time=0.001000
  EtherCAT PDO Transmit22 : slrealtimeethercatlib/EtherCAT PDO Transmit  Priority=3  sig_name=Device_01 (BCE12-0605).Rx_Cell_11.setCurrent  sig_offset=760  sig_type=single  type_size=32  sig_dim=1  device_id=0  sample_time=0.001000
  EtherCAT PDO Transmit23 : slrealtimeethercatlib/EtherCAT PDO Transmit  Priority=3  sig_name=Device_01 (BCE12-0605).Rx_Cell_12.setVoltage  sig_offset=800  sig_type=single  type_size=32  sig_dim=1  device_id=0  sample_time=0.001000
  EtherCAT PDO Transmit24 : slrealtimeethercatlib/EtherCAT PDO Transmit  Priority=3  sig_name=Device_01 (BCE12-0605).Rx_Cell_12.setCurrent  sig_offset=832  sig_type=single  type_size=32  sig_dim=1  device_id=0  sample_time=0.001000
  EtherCAT PDO Transmit25 : slrealtimeethercatlib/EtherCAT PDO Transmit  Priority=3  sig_name=Device_01 (BCE12-0605).Rx_Cell_10.enableCell  sig_offset=648  sig_type=uint8  type_size=8  sig_dim=1  device_id=0  sample_time=0.001000
  EtherCAT PDO Transmit26 : slrealtimeethercatlib/EtherCAT PDO Transmit  Priority=3  sig_name=Device_01 (BCE12-0605).Rx_Cell_11.enableCell  sig_offset=720  sig_type=uint8  type_size=8  sig_dim=1  device_id=0  sample_time=0.001000
  EtherCAT PDO Transmit27 : slrealtimeethercatlib/EtherCAT PDO Transmit  Priority=3  sig_name=Device_01 (BCE12-0605).Rx_Cell_12.enableCell  sig_offset=792  sig_type=uint8  type_size=8  sig_dim=1  device_id=0  sample_time=0.001000
  EtherCAT PDO Transmit3 : slrealtimeethercatlib/EtherCAT PDO Transmit  Priority=3  sig_name=Device_01 (BCE12-0605).Rx_Cell_03.enableCell  sig_offset=144  sig_type=uint8  type_size=8  sig_dim=1  device_id=0  sample_time=0.001000
  EtherCAT PDO Transmit4 : slrealtimeethercatlib/EtherCAT PDO Transmit  Priority=3  sig_name=Device_01 (BCE12-0605).Rx_Cell_04.enableCell  sig_offset=216  sig_type=uint8  type_size=8  sig_dim=1  device_id=0  sample_time=0.001000
  EtherCAT PDO Transmit5 : slrealtimeethercatlib/EtherCAT PDO Transmit  Priority=3  sig_name=Device_01 (BCE12-0605).Rx_Cell_05.enableCell  sig_offset=288  sig_type=uint8  type_size=8  sig_dim=1  device_id=0  sample_time=0.001000
  EtherCAT PDO Transmit6 : slrealtimeethercatlib/EtherCAT PDO Transmit  Priority=3  sig_name=Device_01 (BCE12-0605).Rx_Cell_06.enableCell  sig_offset=360  sig_type=uint8  type_size=8  sig_dim=1  device_id=0  sample_time=0.001000
  EtherCAT PDO Transmit7 : slrealtimeethercatlib/EtherCAT PDO Transmit  Priority=3  sig_name=Device_01 (BCE12-0605).Rx_Cell_07.enableCell  sig_offset=432  sig_type=uint8  type_size=8  sig_dim=1  device_id=0  sample_time=0.001000
  EtherCAT PDO Transmit8 : slrealtimeethercatlib/EtherCAT PDO Transmit  Priority=3  sig_name=Device_01 (BCE12-0605).Rx_Cell_08.enableCell  sig_offset=504  sig_type=uint8  type_size=8  sig_dim=1  device_id=0  sample_time=0.001000
  EtherCAT PDO Transmit9 : slrealtimeethercatlib/EtherCAT PDO Transmit  Priority=3  sig_name=Device_01 (BCE12-0605).Rx_Cell_09.enableCell  sig_offset=576  sig_type=uint8  type_size=8  sig_dim=1  device_id=0  sample_time=0.001000
  Get SubDevice State : slrealtimeethercatlib/Get SubDevice State  device_id=0  subdevice_name=Device_01 (BCE12-0605)  sample_time=0.001  subdevice_addr=1001  selected_subdevice=Term 1 (EK1100)  timeout=500  subdevice_found=1
  Logical Operator{,1..11} (12 alike) : Logic  AllPortsSameDT=off  OutDataTypeStr=boolean
  Saturation Dynamic{,1..11} (12 alike) : simulink/Discontinuities/Saturation Dynamic  OutMin=[]  OutMax=[]  OutDataTypeStr=Inherit: Same as second input  OutDataType=fixdt(1, 16)  OutScaling=2^-10  DoSatur=off
  Set SubDevice State : slrealtimeethercatlib/Set SubDevice State  device_id=0  subdevice_name=Device_01 (BCE12-0605)  sample_time=0.001  subdevice_addr=1001  selected_subdevice=Term 1 (EK1100)  subdevice_found=1
  Terminator1 : Terminator
  Terminator2 : Terminator
  wires:
  Logical Operator11/1 -> Data Type Conversion12/1
  Bus Selector12/1 -> Logical Operator11/2  "<Enable>"
  Logical Operator10/1 -> Data Type Conversion11/1
  Bus Selector11/1 -> Logical Operator10/2  "<Enable>"
  Logical Operator9/1 -> Data Type Conversion10/1
  Bus Selector10/1 -> Logical Operator9/2  "<Enable>"
  Logical Operator8/1 -> Data Type Conversion9/1
  Bus Selector9/1 -> Logical Operator8/2  "<Enable>"
  Logical Operator7/1 -> Data Type Conversion8/1
  Bus Selector8/1 -> Logical Operator7/2  "<Enable>"
  Logical Operator6/1 -> Data Type Conversion7/1
  Bus Selector7/1 -> Logical Operator6/2  "<Enable>"
  Logical Operator5/1 -> Data Type Conversion6/1
  Bus Selector6/1 -> Logical Operator5/2  "<Enable>"
  Logical Operator4/1 -> Data Type Conversion5/1
  Bus Selector5/1 -> Logical Operator4/2  "<Enable>"
  Logical Operator3/1 -> Data Type Conversion4/1
  Bus Selector4/1 -> Logical Operator3/2  "<Enable>"
  Logical Operator2/1 -> Data Type Conversion3/1
  Bus Selector3/1 -> Logical Operator2/2  "<Enable>"
  Logical Operator1/1 -> Data Type Conversion2/1
  Bus Selector2/1 -> Logical Operator1/2  "<Enable>"
  Logical Operator/1 -> Data Type Conversion1/1
  Bus Selector1/1 -> Logical Operator/2  "<Enable>"
  CellEnableDelay/1 -> Logical Operator/1, Logical Operator1/1, Logical Operator2/1, Logical Operator3/1, Logical Operator4/1, Logical Operator5/1, Logical Operator6/1, Logical Operator7/1, Logical Operator8/1, Logical Operator9/1, Logical Operator10/1, Logical Operator11/1
  Constant12/1 -> Set SubDevice State/1
  Compare To Constant25/1 -> Set SubDevice State/2
  Set SubDevice State/1 -> Terminator1/1
  Set SubDevice State/2 -> Terminator2/1
  Get SubDevice State/1 -> Compare To Constant25/1
  Saturation Dynamic11/1 -> EtherCAT PDO Transmit23/1
  Constant11/1 -> Saturation Dynamic11/3
  Saturation Dynamic10/1 -> EtherCAT PDO Transmit21/1
  Constant10/1 -> Saturation Dynamic10/3
  Saturation Dynamic9/1 -> EtherCAT PDO Transmit19/1
  Constant9/1 -> Saturation Dynamic9/3
  Saturation Dynamic8/1 -> EtherCAT PDO Transmit17/1
  Constant8/1 -> Saturation Dynamic8/3
  Saturation Dynamic7/1 -> EtherCAT PDO Transmit15/1
  Constant7/1 -> Saturation Dynamic7/3
  Saturation Dynamic6/1 -> EtherCAT PDO Transmit13/1
  Constant6/1 -> Saturation Dynamic6/3
  Saturation Dynamic5/1 -> EtherCAT PDO Transmit11/1
  Constant5/1 -> Saturation Dynamic5/3
  Saturation Dynamic4/1 -> EtherCAT PDO Transmit09/1
  Constant4/1 -> Saturation Dynamic4/3
  Saturation Dynamic3/1 -> EtherCAT PDO Transmit07/1
  Constant3/1 -> Saturation Dynamic3/3
  Saturation Dynamic2/1 -> EtherCAT PDO Transmit05/1
  Constant2/1 -> Saturation Dynamic2/3
  Saturation Dynamic1/1 -> EtherCAT PDO Transmit03/1
  Constant1/1 -> Saturation Dynamic1/3
  BceVoltageLimit/1 -> Saturation Dynamic1/1, Saturation Dynamic2/1, Saturation Dynamic3/1, Saturation Dynamic4/1, Saturation Dynamic5/1, Saturation Dynamic6/1, Saturation Dynamic7/1, Saturation Dynamic8/1, Saturation Dynamic9/1, Saturation Dynamic10/1, Saturation Dynamic11/1, Saturation Dynamic/1
  Constant/1 -> Saturation Dynamic/3
  Saturation Dynamic/1 -> EtherCAT PDO Transmit01/1
  Bus Selector6/3 -> EtherCAT PDO Transmit12/1  "<I>"
  Bus Selector/4 -> Bus Selector4/1  "<Cell_4>"
  Data Type Conversion7/1 -> EtherCAT PDO Transmit7/1
  Bus Selector11/3 -> EtherCAT PDO Transmit22/1  "<I>"
  Bus Selector9/3 -> EtherCAT PDO Transmit18/1  "<I>"
  Bus Selector/8 -> Bus Selector8/1  "<Cell_8>"
  Bus Selector8/2 -> Saturation Dynamic7/2  "<V>"
  Bus Selector5/2 -> Saturation Dynamic4/2  "<V>"
  Data Type Conversion11/1 -> EtherCAT PDO Transmit26/1
  Bus Selector5/3 -> EtherCAT PDO Transmit10/1  "<I>"
  Data/1 -> Bus Selector/1
  Bus Selector10/3 -> EtherCAT PDO Transmit20/1  "<I>"
  Bus Selector/11 -> Bus Selector11/1  "<Cell_11>"
  Bus Selector3/2 -> Saturation Dynamic2/2  "<V>"
  Bus Selector2/3 -> EtherCAT PDO Transmit04/1  "<I>"
  Bus Selector10/2 -> Saturation Dynamic9/2  "<V>"
  Bus Selector12/3 -> EtherCAT PDO Transmit24/1  "<I>"
  Bus Selector/5 -> Bus Selector5/1  "<Cell_5>"
  Bus Selector/10 -> Bus Selector10/1  "<Cell_10>"
  Bus Selector1/3 -> EtherCAT PDO Transmit02/1  "<I>"
  Data Type Conversion3/1 -> EtherCAT PDO Transmit3/1
  Bus Selector4/2 -> Saturation Dynamic3/2  "<V>"
  Bus Selector6/2 -> Saturation Dynamic5/2  "<V>"
  Bus Selector3/3 -> EtherCAT PDO Transmit06/1  "<I>"
  Bus Selector/12 -> Bus Selector12/1  "<Cell_12>"
  Bus Selector4/3 -> EtherCAT PDO Transmit08/1  "<I>"
  Data Type Conversion1/1 -> EtherCAT PDO Transmit1/1
  Data Type Conversion10/1 -> EtherCAT PDO Transmit25/1
  Data Type Conversion12/1 -> EtherCAT PDO Transmit27/1
  Data Type Conversion5/1 -> EtherCAT PDO Transmit5/1
  Data Type Conversion9/1 -> EtherCAT PDO Transmit9/1
  Data Type Conversion6/1 -> EtherCAT PDO Transmit6/1
  Data Type Conversion4/1 -> EtherCAT PDO Transmit4/1
  Bus Selector/9 -> Bus Selector9/1  "<Cell_9>"
  Bus Selector7/3 -> EtherCAT PDO Transmit14/1  "<I>"
  Bus Selector7/2 -> Saturation Dynamic6/2  "<V>"
  Data Type Conversion2/1 -> EtherCAT PDO Transmit2/1
  Bus Selector/6 -> Bus Selector6/1  "<Cell_6>"
  Bus Selector/2 -> Bus Selector2/1  "<Cell_2>"
  Bus Selector1/2 -> Saturation Dynamic/2  "<V>"
  Bus Selector/3 -> Bus Selector3/1  "<Cell_3>"
  Bus Selector8/3 -> EtherCAT PDO Transmit16/1  "<I>"
  Bus Selector/1 -> Bus Selector1/1  "<Cell_1>"
  Bus Selector11/2 -> Saturation Dynamic10/2  "<V>"
  Bus Selector/7 -> Bus Selector7/1  "<Cell_7>"
  Bus Selector2/2 -> Saturation Dynamic1/2  "<V>"
  Bus Selector12/2 -> Saturation Dynamic11/2  "<V>"
  Bus Selector9/2 -> Saturation Dynamic8/2  "<V>"
  Data Type Conversion8/1 -> EtherCAT PDO Transmit8/1
